simulink subsystem "PieroModelado"  (R2023b)
settings: Solver=VariableStepAuto  StartTime=0.0  StopTime=10.0  RelTol=1e-3
settings Model: Creator=Usuario  LastModifiedBy=Usuario

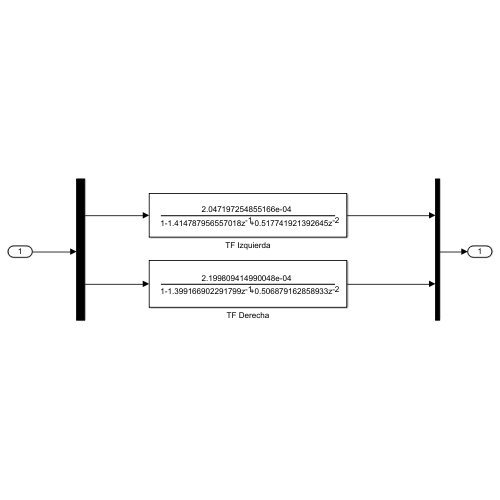
[thumbnail: Simulink's stored preview of the top-level diagram]
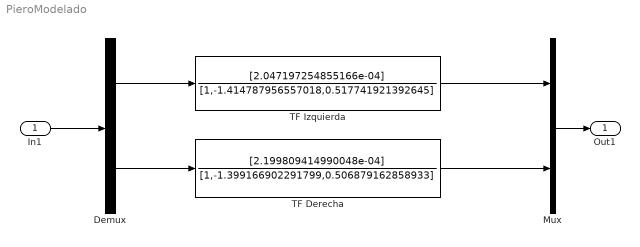
== system PieroModelado ==
  In1 : Inport
  Demux : Demux  Outputs=2
  Mux : Mux  Inputs=2
  TF Derecha : DiscreteFilter  Numerator=[2.199809414990048e-04]  Denominator=[1,-1.399166902291799,0.506879162858933]
  TF Izquierda : DiscreteFilter  Numerator=[2.047197254855166e-04]  Denominator=[1,-1.414787956557018,0.517741921392645]
  Out1 : Outport
  wires:
  TF Derecha/1 -> Mux/2
  Demux/1 -> TF Izquierda/1
  Demux/2 -> TF Derecha/1
  In1/1 -> Demux/1
  TF Izquierda/1 -> Mux/1
  Mux/1 -> Out1/1
